simulink subsystem "Driver"  (R2023b)
settings: Solver=VariableStepAuto  StartTime=0.0  StopTime=10.0  RelTol=1e-3
undefined symbols (not defined in the file): BDrive, BStartSwitch, IConstantStep, INissanLeaf, ITest, NProfile, tConstantStep, tSim
settings Model: Creator=Elio  LastModifiedBy=Elio

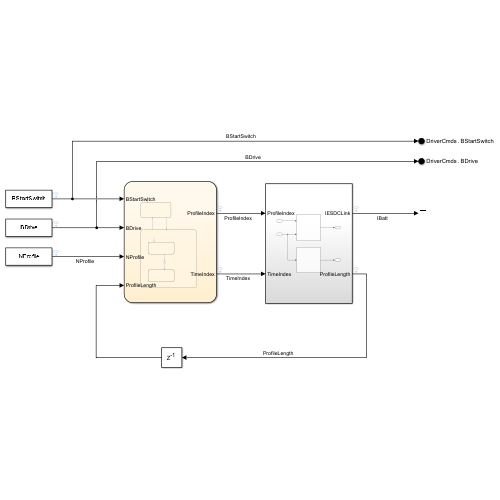
[thumbnail: Simulink's stored preview of the top-level diagram]
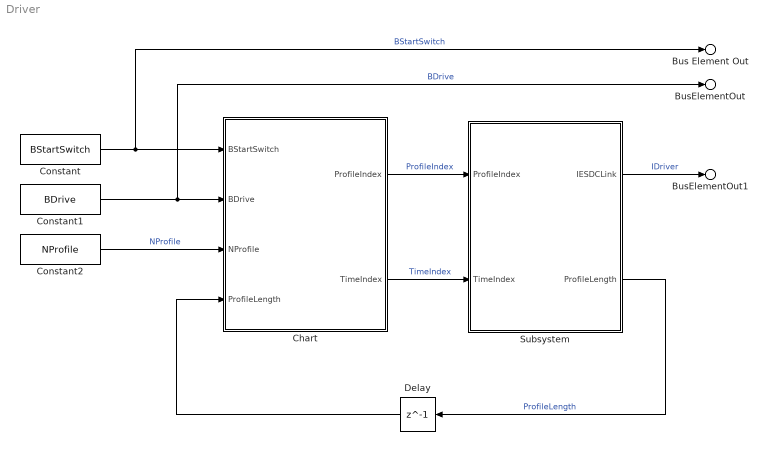
== system Driver ==
  Chart : Stateflow chart  TreatAsAtomicUnit=on
      settings: PortSchema="{\"entries\":[{\"content\":{\"sides\":[{\"content\":{\"connectorIds\":[\"In2\",\"In1\",\"In4\",\"In3\"]},\"type\":\"ConnectorPlacement.EquallySpacedRectSide\",\"uuid\":\"6ea83b0b-0330-48d9-9645-eb63bf4ae346\"},{\"content\":{\"connectorIds\":[\"Out2\",\"Out1\"],\"side\":\"RIGHT\"},\"type\":\"ConnectorPlacement.EquallySpacedRectSide\",\"uuid\":\"65706aaf-4f6b-45f1-81e0-083514d97b7c\"},{\"content\":{\"side\":\"TOP\"},\"type\":\"ConnectorPlacement.EquallySpacedRectSide\",\"uuid\":\"23c5670b-958f-42b6-b08d-f5741aaf4b2a\"}]},\"type\":\"ConnectorPlacement.EquallySpacedConnector\",\"uuid\":\"68ad297d-9b0b-49a6-94c0-e696e07492cf\"}],\"packageUris\":[\"http://schema.mathworks.com/mf0/Connector/R2020b\"],\"version\":\"1.0\"}"
  Constant : Constant  Value=BStartSwitch  SampleTime=tSim
  Constant1 : Constant  Value=BDrive  SampleTime=tSim
  Constant2 : Constant  Value=NProfile  SampleTime=tSim
  Delay : Delay  DelayLength=1
  Subsystem : Subsystem
  Bus Element Out : Outport  PortName=DriverCmds  Element=BStartSwitch
  BusElementOut : Outport  PortName=DriverCmds  Element=BDrive
  BusElementOut1 : Outport  PortName=DriverCmds  Element=IESDCLink
  wires:
  Subsystem/1(IESDCLink) -> BusElementOut1/1  "IDriver"
  Constant2/1 -> Chart/4(NProfile)  "NProfile"
  Constant/1 -> Bus Element Out/1, Chart/2(BStartSwitch)  "BStartSwitch"
  Delay/1 -> Chart/3(ProfileLength)
  Constant1/1 -> BusElementOut/1, Chart/1(BDrive)  "BDrive"
  Chart/2(ProfileIndex) -> Subsystem/1(ProfileIndex)  "ProfileIndex"
  Subsystem/2(ProfileLength) -> Delay/1  "ProfileLength"
  Chart/1(TimeIndex) -> Subsystem/2(TimeIndex)  "TimeIndex"

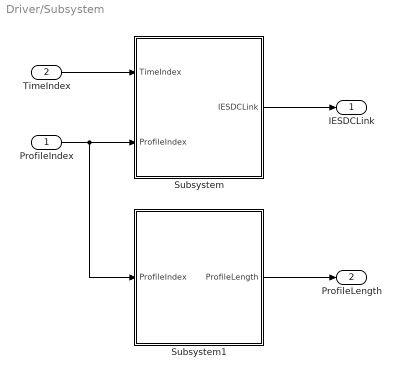
== system Driver/Subsystem ==
  ProfileIndex : Inport
  TimeIndex : Inport  Port=2
  Subsystem : Subsystem
  Subsystem1 : Subsystem
  IESDCLink : Outport
  ProfileLength : Outport  Port=2
  wires:
  Subsystem/1(IESDCLink) -> IESDCLink/1
  TimeIndex/1 -> Subsystem/1(TimeIndex)
  ProfileIndex/1 -> Subsystem1/1(ProfileIndex), Subsystem/2(ProfileIndex)
  Subsystem1/1(ProfileLength) -> ProfileLength/1

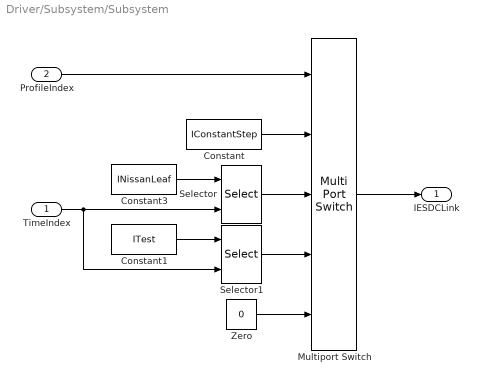
== system Driver/Subsystem/Subsystem ==
  TimeIndex : Inport
  ProfileIndex : Inport  Port=2
  Constant : Constant  Value=IConstantStep  SampleTime=tSim
  Constant1 : Constant  Value=ITest  SampleTime=tSim
  Constant3 : Constant  Value=INissanLeaf  SampleTime=tSim
  Multiport Switch : MultiPortSwitch  Inputs=4  DiagnosticForDefault=None  SaturateOnIntegerOverflow=off  InputSameDT=off
  Selector : Selector  InputPortWidth=4609901  IndexOptions=Index vector (port)  Indices=[1 3]  OutputSizes=1
  Selector1 : Selector  InputPortWidth=10  IndexOptions=Index vector (port)  Indices=[1 3]  OutputSizes=1
  Zero : Constant  Value=0  OutDataTypeStr=Inherit: Inherit via back propagation
  IESDCLink : Outport
  wires:
  Constant/1 -> Multiport Switch/2
  Selector/1 -> Multiport Switch/3
  Selector1/1 -> Multiport Switch/4
  ProfileIndex/1 -> Multiport Switch/1
  Multiport Switch/1 -> IESDCLink/1
  Constant3/1 -> Selector/1
  Zero/1 -> Multiport Switch/5
  Constant1/1 -> Selector1/1
  TimeIndex/1 -> Selector1/2, Selector/2

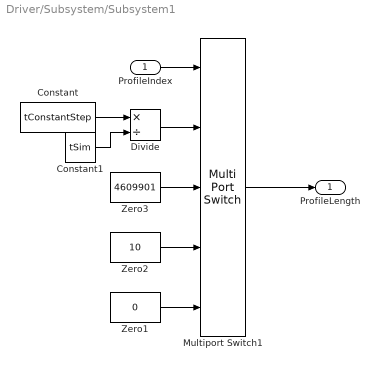
== system Driver/Subsystem/Subsystem1 ==
  ProfileIndex : Inport
  Constant : Constant  Value=tConstantStep  SampleTime=tSim
  Constant1 : Constant  Value=tSim  SampleTime=tSim
  Divide : Product  Inputs=*/
  Multiport Switch1 : MultiPortSwitch  Inputs=4  DiagnosticForDefault=None  SaturateOnIntegerOverflow=off  InputSameDT=off
  Zero1 : Constant  Value=0  OutDataTypeStr=Inherit: Inherit via back propagation
  Zero2 : Constant  Value=10  OutDataTypeStr=Inherit: Inherit via back propagation
  Zero3 : Constant  Value=4609901  OutDataTypeStr=Inherit: Inherit via back propagation
  ProfileLength : Outport
  wires:
  Divide/1 -> Multiport Switch1/2
  Constant1/1 -> Divide/2
  Constant/1 -> Divide/1
  Zero3/1 -> Multiport Switch1/3
  Zero2/1 -> Multiport Switch1/4
  Zero1/1 -> Multiport Switch1/5
  Multiport Switch1/1 -> ProfileLength/1
  ProfileIndex/1 -> Multiport Switch1/1

== stateflow chart Driver/Chart ==
  state STOP
    entry:
    ProfileIndex = 0;
    TimeIndex = 1;
  state STANDBY
  state RUN_PROFILE
    state INCREMENT
      entry:
      ProfileIndex = NProfile;
    state DONE
      entry:
      ProfileIndex = 0;
    (default) -> INCREMENT
    INCREMENT -> (junction 11) : {TimeIndex += 1;}
    (junction 11) -> DONE : [TimeIndex > ProfileLength]
  (default) -> STOP
  RUN_PROFILE -> STOP : [!BStartSwitch || !BDrive || (NProfile==0)]
  STOP -> STANDBY : [BStartSwitch && BDrive && (NProfile==0)]
  STANDBY -> RUN_PROFILE : [NProfile!=0]
  data: BDrive input boolean; BStartSwitch input boolean; ProfileLength input; TimeIndex output double; ProfileIndex output double; NProfile input
